simulink model "E_Platoon"  (R2025b)
settings: Solver=FixedStepAuto  StartTime=0.0  StopTime=inf  FixedStep=0.1  RelTol=1e-3
values from neighbouring files (symbols this model uses):
  Battery_Capacity = [1,4500]    [EV_Truck.m]
  battery_SOC_resistance = battery_SOC(:,3)    [EV_Truck.m]
  battery_SOC_SOC = battery_SOC(:,1)    [EV_Truck.m]
  battery_SOC_voltage = battery_SOC(:,2)    [EV_Truck.m]
  motor_efficiency_efficiency = table2array(motor_efficiency(2:height(motor_efficiency),2:width(motor_efficiency)))    [EV_Truck.m]
  motor_efficiency_RPM = table2array(motor_efficiency(2:height(motor_efficiency),1))    [EV_Truck.m]
  motor_efficiency_torque = transpose(motor_efficiency_torque)    [EV_Truck.m]
  motor_RPM_torque = table2array(motor_torque(1:14,1))    [EV_Truck.m]
  motor_torque_RPM = table2array(motor_torque(1:14,2))    [EV_Truck.m]
undefined symbols (not defined in the file or in its folder): Battery_Initial_SOC, DiscIntNeverNeededParam
libraries: simulink x8, BatteryEstimators x4, mpcadaslib x2, slpidlib x2
(part 1 of 2)
settings Model: Creator=geunu6319  LastModifiedBy=geunu6319
settings DataIOCC: SaveFormat=Array  ReturnWorkspaceOutputs=off

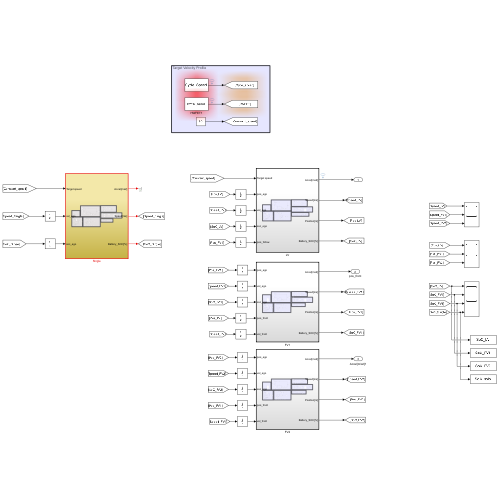
[thumbnail: Simulink's stored preview of the top-level diagram]
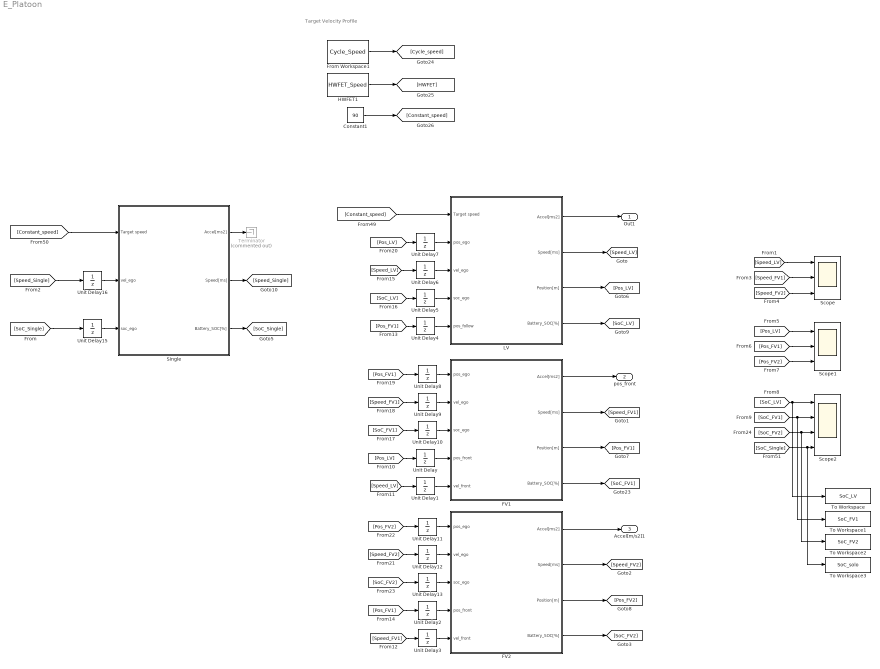
== system E_Platoon ==
  note: Target Velocity Profile
  Constant1 : Constant  Value=90  SampleTime=0
  FV1 : Subsystem  TreatAsAtomicUnit=on
  FV2 : Subsystem  TreatAsAtomicUnit=on
  From Workspace1 : FromWorkspace  VariableName=Cycle_Speed  SampleTime=-1
  HWFET1 : FromWorkspace  VariableName=HWFET_Speed  SampleTime=-1
  LV : Subsystem  TreatAsAtomicUnit=on
  Scope : Scope  NumInputPorts=3
      settings: ActiveDisplayYMinimum=-3.56247  ActiveDisplayYMaximum=3.7997  DataLoggingVariableName=ScopeData5
  Scope1 : Scope  NumInputPorts=3
      settings: ActiveDisplayYMinimum=-50980.76527  ActiveDisplayYMaximum=458458.14542  DataLoggingVariableName=ScopeData6
  Scope2 : Scope  NumInputPorts=4
      settings: ActiveDisplayYMinimum=88.74997  ActiveDisplayYMaximum=101.25001
  Single : Subsystem  TreatAsAtomicUnit=on
  Terminator : Terminator  Commented=on
  To Workspace : ToWorkspace  VariableName=SoC_LV  SaveFormat=Timeseries  SampleTime=-1
  To Workspace1 : ToWorkspace  VariableName=SoC_FV1  SaveFormat=Timeseries  SampleTime=-1
  To Workspace2 : ToWorkspace  VariableName=SoC_FV2  SaveFormat=Timeseries  SampleTime=-1
  To Workspace3 : ToWorkspace  VariableName=SoC_solo  SaveFormat=Timeseries  SampleTime=-1
  Unit Delay{,1..13,15..16} (16 alike) : UnitDelay  SampleTime=-1  HasFrameUpgradeWarning=on
  Out1 : Outport
  pos_front : Outport  Port=2
  Accel[m/s2]1 : Outport  Port=3
  wires:
  LV/2(Speed[ms]) -> [Speed_LV]
  [Pos_LV] -> Scope1/1
  Unit Delay2/1 -> FV2/4(pos_front)
  Unit Delay5/1 -> LV/4(soc_ego)
  [SoC_FV1] -> Unit Delay10/1
  [Speed_LV] -> Unit Delay1/1
  Unit Delay15/1 -> Single/3(soc_ego)
  FV1/1(Accel[ms2]) -> pos_front/1
  [Speed_LV] -> Scope/1
  [SoC_Single] -> To Workspace3/1, Scope2/4
  LV/4(Battery_SOC[%]) -> [SoC_LV]
  Single/1(Accel[ms2]) -> Terminator/1
  [Speed_FV1] -> Unit Delay3/1
  [Constant_speed] -> LV/1(Target speed)
  [Pos_FV1] -> Scope1/2
  Unit Delay16/1 -> Single/2(vel_ego)
  [Pos_LV] -> Unit Delay7/1
  [SoC_FV2] -> To Workspace2/1, Scope2/3
  Constant1/1 -> [Constant_speed]
  Unit Delay6/1 -> LV/3(vel_ego)
  Unit Delay3/1 -> FV2/5(vel_front)
  [Speed_FV1] -> Scope/2
  [Speed_FV2] -> Unit Delay12/1
  Unit Delay11/1 -> FV2/1(pos_ego)
  FV2/4(Battery_SOC[%]) -> [SoC_FV2]
  FV2/2(Speed[ms]) -> [Speed_FV2]
  [Speed_Single] -> Unit Delay16/1
  FV2/3(Position[m]) -> [Pos_FV2]
  [SoC_Single] -> Unit Delay15/1
  Unit Delay12/1 -> FV2/2(vel_ego)
  [Pos_FV2] -> Unit Delay11/1
  Unit Delay4/1 -> LV/5(pos_follow)
  LV/3(Position[m]) -> [Pos_LV]
  [Speed_FV2] -> Scope/3
  Unit Delay13/1 -> FV2/3(soc_ego)
  Unit Delay1/1 -> FV1/5(vel_front)
  [Speed_LV] -> Unit Delay6/1
  [Speed_FV1] -> Unit Delay9/1
  FV2/1(Accel[ms2]) -> Accel[m/s2]1/1
  From Workspace1/1 -> [Cycle_speed]
  [Pos_FV1] -> Unit Delay4/1
  FV1/4(Battery_SOC[%]) -> [SoC_FV1]
  LV/1(Accel[ms2]) -> Out1/1
  [Pos_LV] -> Unit Delay/1
  [SoC_LV] -> To Workspace/1, Scope2/1
  FV1/3(Position[m]) -> [Pos_FV1]
  Single/2(Speed[ms]) -> [Speed_Single]
  [Pos_FV2] -> Scope1/3
  Single/3(Battery_SOC[%]) -> [SoC_Single]
  Unit Delay9/1 -> FV1/2(vel_ego)
  [Pos_FV1] -> Unit Delay2/1
  Unit Delay8/1 -> FV1/1(pos_ego)
  [Pos_FV1] -> Unit Delay8/1
  HWFET1/1 -> [HWFET]
  Unit Delay10/1 -> FV1/3(soc_ego)
  [SoC_FV2] -> Unit Delay13/1
  Unit Delay7/1 -> LV/2(pos_ego)
  [Constant_speed] -> Single/1(Target speed)
  [SoC_FV1] -> To Workspace1/1, Scope2/2
  Unit Delay/1 -> FV1/4(pos_front)
  [SoC_LV] -> Unit Delay5/1
  FV1/2(Speed[ms]) -> [Speed_FV1]

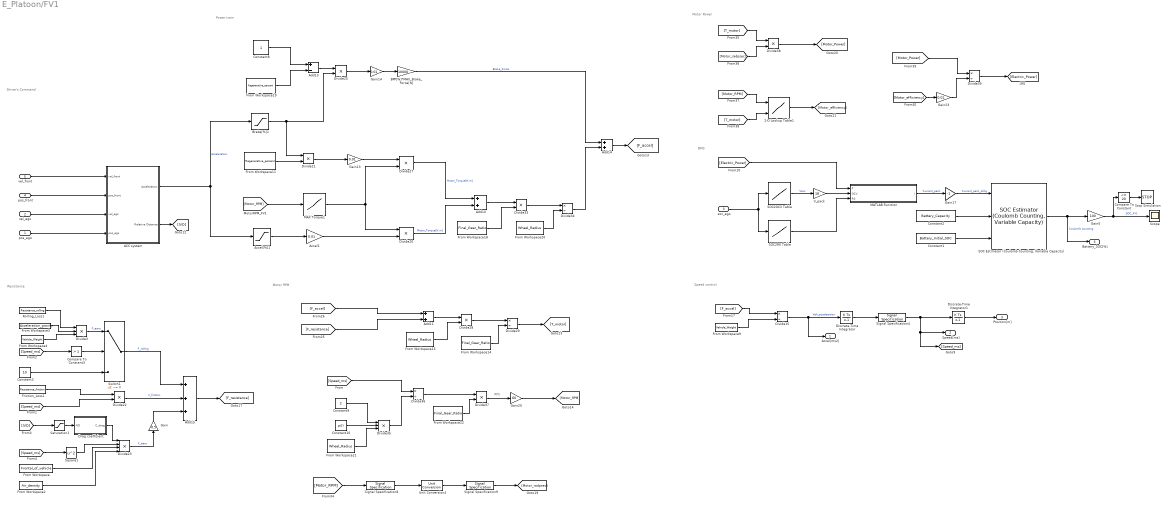
== system E_Platoon/FV1 ==
  note: Driver's Command
  note: Motor RPM
  note: Motor Power
  note: Power train
  note: RPS
  note: Resistance
  note: Speed control
  note: BMS
  pos_ego : Inport
  vel_ego : Inport  Port=2
  soc_ego : Inport  Port=3
  pos_front : Inport  Port=4
  vel_front : Inport  Port=5
  2-D Lookup Table1 : Lookup_n-D  BreakpointsForDimension1=motor_efficiency_RPM  BreakpointsForDimension2=motor_efficiency_torque  Table=motor_efficiency_efficiency  RemoveProtectionInput=on  InternalRulePriority=Speed  RndMeth=Simplest
      settings: InputPortMap=u0,u1
  ACC system : Subsystem
  Accel1 : Gain  Gain=0.01
  Accel[%]1 : Saturate  UpperLimit=100  LowerLimit=0
  Add10 : Sum
  Add11 : Sum
  Add13 : Sum  Inputs=+-
  Add14 : Sum
  Add15 : Sum  Inputs=+++
  BPP[%]*MAX_Brake_Force[N] : Gain  Gain=10000
  Brake[%]1 : Saturate  UpperLimit=0  LowerLimit=-100
  Compare To Constant : simulink/Logic and Bit Operations/Compare To Constant  relop=<=  const=20  OutDataTypeStr=boolean
  Compare To Constant3 : simulink/Logic and Bit Operations/Compare To Constant  relop=>  const=1  OutDataTypeStr=boolean
  Constant1 : Constant  Value=Battery_Initial_SOC
  Constant10 : Constant  Value=pi()
  Constant2 : Constant  Value=Battery_Capacity
  Constant3 : Constant  Value=10
  Constant8 : Constant
  Constant9 : Constant  Value=2
  Discrete-Time Integrator : DiscreteIntegrator  SampleTime=-1  ICPrevOutput=DiscIntNeverNeededParam  ICPrevScaledInput=DiscIntNeverNeededParam
  Discrete-Time Integrator1 : DiscreteIntegrator  SampleTime=-1  ICPrevOutput=DiscIntNeverNeededParam  ICPrevScaledInput=DiscIntNeverNeededParam
  Divide{15,29,34,36,39} (5 alike) : Product  Inputs=*/
  Divide{20..22,25,27..28,33,37..38} (9 alike) : Product  Inputs=**
  Divide23 : Product  Inputs=****
  Divide3 : Product  Inputs=***
  Divide35 : Product  Inputs=***
  Drag coefficient : MATLAB Function  TreatAsAtomicUnit=on
  Friction_Loss1 : FromWorkspace  VariableName=Resistance_friction  SampleTime=0.01
  From Workspace : FromWorkspace  VariableName=Frontal_of_vehicle  SampleTime=0.01
  From Workspace11 : FromWorkspace  VariableName=Regenerative_percent  SampleTime=0.01
  From Workspace14 : FromWorkspace  VariableName=Final_Gear_Ratio  SampleTime=0.01
  From Workspace15 : FromWorkspace  VariableName=Wheel_Radius  SampleTime=0.01
  From Workspace18 : FromWorkspace  VariableName=Final_Gear_Ratio  SampleTime=0.01
  From Workspace19 : FromWorkspace  VariableName=Regenerative_percent  SampleTime=0.01
  From Workspace2 : FromWorkspace  VariableName=Air_density  SampleTime=0.01
  From Workspace20 : FromWorkspace  VariableName=Wheel_Radius  SampleTime=0.01
  From Workspace21 : FromWorkspace  VariableName=Wheel_Radius  SampleTime=0.01
  From Workspace22 : FromWorkspace  VariableName=Final_Gear_Ratio  SampleTime=0.01
  From Workspace3 : FromWorkspace  VariableName=Acceleration_gravity  SampleTime=0.01
  From Workspace4 : FromWorkspace  VariableName=Vehicle_Weight  SampleTime=0.01
  From Workspace9 : FromWorkspace  VariableName=Vehicle_Weight  SampleTime=0.01
  Gain : Gain  Gain=0.5
  Gain13 : Gain  Gain=0.01
  Gain14 : Gain  Gain=0.01
  Gain17 : Gain  Gain=-1
  Gain20 : Gain  Gain=60
  Gain23 : Gain  Gain=0.01
  Gain5 : Gain  Gain=100
  MATLAB Function : MATLAB Function  TreatAsAtomicUnit=on
  MAX Torque1 : Lookup_n-D  NumberOfTableDimensions=1  BreakpointsForDimension1=motor_RPM_torque  Table=motor_torque_RPM  RemoveProtectionInput=on  InternalRulePriority=Speed  RndMeth=Simplest
  Rolling_Loss1 : FromWorkspace  VariableName=Resistance_rolling  SampleTime=0.01
  "SOC Estimator (Coulomb Counting, Variable Capacity)" : BatteryEstimators/SOC Estimator (Coulomb Counting, Variable Capacity)  CurrentInputPartition=on  Ts=1  DataType=Inherit: auto
      settings: LibrarySourceBlock=|
      | batt_sl_lib/Estimators/SOC Estimator
      | (Coulomb Counting, Variable Capacity)
  SOC2OCV Table : Lookup_n-D  NumberOfTableDimensions=1  BreakpointsForDimension1=battery_SOC_SOC  Table=battery_SOC_voltage  ExtrapMethod=Clip  RemoveProtectionInput=on  UseLastTableValue=on  InternalRulePriority=Speed  RndMeth=Simplest
  SOC2R0 Table : Lookup_n-D  NumberOfTableDimensions=1  BreakpointsForDimension1=battery_SOC_SOC  Table=battery_SOC_resistance  RemoveProtectionInput=on  InternalRulePriority=Speed  RndMeth=Simplest
  Saturation1 : Saturate  UpperLimit=100  LowerLimit=0
  Scope : Scope
      settings: DataLoggingVariableName=ScopeData2
  Signal Specification4 : SignalSpecification  Unit=m/s
  Signal Specification8 : SignalSpecification  Unit=rpm
  Signal Specification9 : SignalSpecification  Unit=rad/s
  Square1 : Math  Operator=square
  Stop Simulation : Stop
  Switch1 : Switch  Criteria=u2 ~= 0  SaturateOnIntegerOverflow=off  InputSameDT=off
  Unit Conversion4 : UnitConversion
  V_pack : Gain  Gain=18
  Accel[ms2] : Outport
  Speed[ms] : Outport  Port=2
  Position[m] : Outport  Port=3
  Battery_SOC[%] : Outport  Port=4
  wires:
  vel_front/1 -> ACC system/1(vel_front)
  pos_front/1 -> ACC system/2(pos_front)
  ACC system/2(Relative Distance) -> [IVD]
  From Workspace15/1 -> Divide28/2
  Divide28/1 -> Divide29/1
  From Workspace14/1 -> Divide29/2
  Divide37/1 -> Gain20/1
  Divide36/1 -> Divide37/1
  From Workspace21/1 -> Divide35/3
  Add10/1 -> Divide33/1
  Unit Conversion4/1 -> Signal Specification9/1
  Gain14/1 -> BPP[%]*MAX_Brake_Force[N]/1
  Signal Specification9/1 -> [Motor_radpsec]
  MAX Torque1/1 -> Divide27/2, Divide20/1
  [Motor_RPM] -> MAX Torque1/1
  Divide35/1 -> Divide36/2
  [Motor_RPM] -> Signal Specification8/1
  Gain13/1 -> Divide27/1
  Divide39/1 -> [Electric_Power]
  Divide34/1 -> Add14/2
  Accel[%]1/1 -> Accel1/1
  [Motor_efficiency] -> Gain23/1
  Brake[%]1/1 -> Divide25/2, Divide21/1
  [Motor_RPM] -> 2-D Lookup Table1/1
  Divide25/1 -> Gain14/1
  Constant9/1 -> Divide35/1
  Add13/1 -> Divide25/1
  Divide20/1 -> Add10/2  "Motor_Torque[N.m]"
  [T_motor] -> Divide38/1
  Divide27/1 -> Add10/1  "Motor_Torque[N.m]"
  Divide33/1 -> Divide34/1
  Add14/1 -> [F_accel]
  From Workspace18/1 -> Divide33/2
  From Workspace20/1 -> Divide34/2
  BPP[%]*MAX_Brake_Force[N]/1 -> Add14/1  "Brake_Force"
  Divide38/1 -> [Motor_Power]
  [F_accel] -> Add11/1
  Constant10/1 -> Divide35/2
  [Motor_Power] -> Divide39/1
  [Motor_radpsec] -> Divide38/2
  Gain20/1 -> [Motor_RPM]
  Divide21/1 -> Gain13/1
  [Speed_ms] -> Divide36/1
  Constant8/1 -> Add13/1
  Signal Specification8/1 -> Unit Conversion4/1
  Accel1/1 -> Divide20/2
  From Workspace19/1 -> Add13/2
  From Workspace11/1 -> Divide21/2
  2-D Lookup Table1/1 -> [Motor_efficiency]
  From Workspace22/1 -> Divide37/2
  Gain23/1 -> Divide39/2
  Divide29/1 -> [T_motor]
  [T_motor] -> 2-D Lookup Table1/2
  Add11/1 -> Divide28/1
  [F_resistance] -> Add11/2
  ACC system/1(Acceleration) -> Accel[%]1/1, Brake[%]1/1  "Acceleration"
  From Workspace3/1 -> Divide3/2
  From Workspace/1 -> Divide23/3
  Gain/1 -> Add15/3
  From Workspace2/1 -> Divide23/4
  Divide3/1 -> Switch1/1  "F_aero"
  Divide23/1 -> Gain/1  "F_aero"
  From Workspace4/1 -> Divide3/3
  Saturation1/1 -> Drag coefficient/1(IVD)
  Add15/1 -> [F_resistance]
  Friction_Loss1/1 -> Divide22/1
  Drag coefficient/1(C_drag) -> Divide23/1
  Rolling_Loss1/1 -> Divide3/1
  Compare To Constant3/1 -> Switch1/2
  Square1/1 -> Divide23/2
  Constant3/1 -> Switch1/3
  [IVD] -> Saturation1/1
  [Speed_ms] -> Square1/1
  [Speed_ms] -> Divide22/2
  [Speed_ms] -> Compare To Constant3/1
  Divide22/1 -> Add15/2  "F_friction"
  Switch1/1 -> Add15/1  "F_rolling"
  pos_ego/1 -> ACC system/4(pos_ego)
  vel_ego/1 -> ACC system/3(vel_ego)
  Signal Specification4/1 -> Discrete-Time Integrator1/1, Speed[ms]/1, [Speed_ms]
  Divide15/1 -> Discrete-Time Integrator/1, Accel[ms2]/1  "Veh_acceleartion"
  From Workspace9/1 -> Divide15/2
  Discrete-Time Integrator1/1 -> Position[m]/1
  [F_accel] -> Divide15/1
  Discrete-Time Integrator/1 -> Signal Specification4/1
  Constant1/1 -> "SOC Estimator (Coulomb Counting, Variable Capacity)"/3
  "SOC Estimator (Coulomb Counting, Variable Capacity)"/1 -> Battery_SOC[%]/1, Gain5/1  "Coulomb counting"
  Constant2/1 -> "SOC Estimator (Coulomb Counting, Variable Capacity)"/2
  MATLAB Function/1(I) -> Gain17/1  "Current_pack"
  soc_ego/1 -> SOC2R0 Table/1, SOC2OCV Table/1
  [Electric_Power] -> MATLAB Function/1(P)
  V_pack/1 -> MATLAB Function/2(OCV)
  Gain17/1 -> "SOC Estimator (Coulomb Counting, Variable Capacity)"/1  "Current_pack_dchg"
  Gain5/1 -> Compare To Constant/1, Scope/1  "SOC_FV1"
  Compare To Constant/1 -> Stop Simulation/1
  SOC2R0 Table/1 -> MATLAB Function/3(R0)
  SOC2OCV Table/1 -> V_pack/1  "Vsoc"

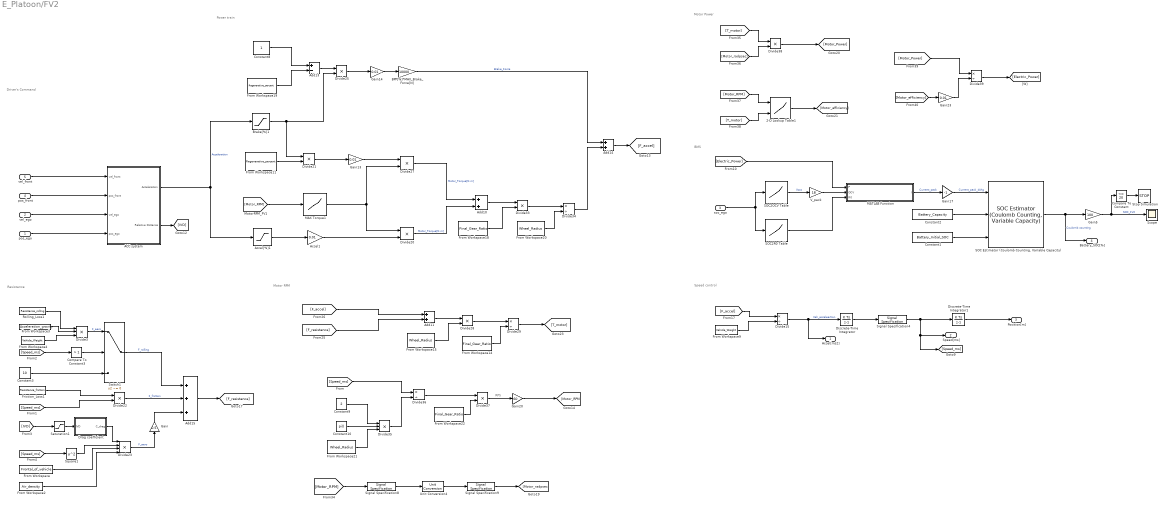
== system E_Platoon/FV2 ==
  note: Driver's Command
  note: Motor RPM
  note: Motor Power
  note: Power train
  note: RPS
  note: Resistance
  note: Speed control
  note: BMS
  pos_ego : Inport
  vel_ego : Inport  Port=2
  soc_ego : Inport  Port=3
  pos_front : Inport  Port=4
  vel_front : Inport  Port=5
  2-D Lookup Table1 : Lookup_n-D  BreakpointsForDimension1=motor_efficiency_RPM  BreakpointsForDimension2=motor_efficiency_torque  Table=motor_efficiency_efficiency  RemoveProtectionInput=on  InternalRulePriority=Speed  RndMeth=Simplest
      settings: InputPortMap=u0,u1
  ACC system : Subsystem
  Accel1 : Gain  Gain=0.01
  Accel[%]1 : Saturate  UpperLimit=100  LowerLimit=0
  Add10 : Sum
  Add11 : Sum
  Add13 : Sum  Inputs=+-
  Add14 : Sum
  Add15 : Sum  Inputs=+++
  BPP[%]*MAX_Brake_Force[N] : Gain  Gain=10000
  Brake[%]1 : Saturate  UpperLimit=0  LowerLimit=-100
  Compare To Constant : simulink/Logic and Bit Operations/Compare To Constant  relop=<=  const=20  OutDataTypeStr=boolean
  Compare To Constant3 : simulink/Logic and Bit Operations/Compare To Constant  relop=>  const=1  OutDataTypeStr=boolean
  Constant1 : Constant  Value=Battery_Initial_SOC
  Constant10 : Constant  Value=pi()
  Constant2 : Constant  Value=Battery_Capacity
  Constant3 : Constant  Value=10
  Constant8 : Constant
  Constant9 : Constant  Value=2
  Discrete-Time Integrator : DiscreteIntegrator  SampleTime=-1  ICPrevOutput=DiscIntNeverNeededParam  ICPrevScaledInput=DiscIntNeverNeededParam
  Discrete-Time Integrator1 : DiscreteIntegrator  SampleTime=-1  ICPrevOutput=DiscIntNeverNeededParam  ICPrevScaledInput=DiscIntNeverNeededParam
  Divide{15,29,34,36,39} (5 alike) : Product  Inputs=*/
  Divide{20..22,25,27..28,33,37..38} (9 alike) : Product  Inputs=**
  Divide23 : Product  Inputs=****
  Divide3 : Product  Inputs=***
  Divide35 : Product  Inputs=***
  Drag coefficient : MATLAB Function  TreatAsAtomicUnit=on
  Friction_Loss1 : FromWorkspace  VariableName=Resistance_friction  SampleTime=0.01
  From Workspace : FromWorkspace  VariableName=Frontal_of_vehicle  SampleTime=0.01
  From Workspace11 : FromWorkspace  VariableName=Regenerative_percent  SampleTime=0.01
  From Workspace14 : FromWorkspace  VariableName=Final_Gear_Ratio  SampleTime=0.01
  From Workspace15 : FromWorkspace  VariableName=Wheel_Radius  SampleTime=0.01
  From Workspace18 : FromWorkspace  VariableName=Final_Gear_Ratio  SampleTime=0.01
  From Workspace19 : FromWorkspace  VariableName=Regenerative_percent  SampleTime=0.01
  From Workspace2 : FromWorkspace  VariableName=Air_density  SampleTime=0.01
  From Workspace20 : FromWorkspace  VariableName=Wheel_Radius  SampleTime=0.01
  From Workspace21 : FromWorkspace  VariableName=Wheel_Radius  SampleTime=0.01
  From Workspace22 : FromWorkspace  VariableName=Final_Gear_Ratio  SampleTime=0.01
  From Workspace3 : FromWorkspace  VariableName=Acceleration_gravity  SampleTime=0.01
  From Workspace4 : FromWorkspace  VariableName=Vehicle_Weight  SampleTime=0.01
  From Workspace9 : FromWorkspace  VariableName=Vehicle_Weight  SampleTime=0.01
  Gain : Gain  Gain=0.5
  Gain13 : Gain  Gain=0.01
  Gain14 : Gain  Gain=0.01
  Gain17 : Gain  Gain=-1
  Gain20 : Gain  Gain=60
  Gain23 : Gain  Gain=0.01
  Gain5 : Gain  Gain=100
  MATLAB Function : MATLAB Function  TreatAsAtomicUnit=on
  MAX Torque1 : Lookup_n-D  NumberOfTableDimensions=1  BreakpointsForDimension1=motor_RPM_torque  Table=motor_torque_RPM  RemoveProtectionInput=on  InternalRulePriority=Speed  RndMeth=Simplest
  Rolling_Loss1 : FromWorkspace  VariableName=Resistance_rolling  SampleTime=0.01
  "SOC Estimator (Coulomb Counting, Variable Capacity)" : BatteryEstimators/SOC Estimator (Coulomb Counting, Variable Capacity)  CurrentInputPartition=on  Ts=1  DataType=Inherit: auto
      settings: LibrarySourceBlock=|
      | batt_sl_lib/Estimators/SOC Estimator
      | (Coulomb Counting, Variable Capacity)
  SOC2OCV Table : Lookup_n-D  NumberOfTableDimensions=1  BreakpointsForDimension1=battery_SOC_SOC  Table=battery_SOC_voltage  ExtrapMethod=Clip  RemoveProtectionInput=on  UseLastTableValue=on  InternalRulePriority=Speed  RndMeth=Simplest
  SOC2R0 Table : Lookup_n-D  NumberOfTableDimensions=1  BreakpointsForDimension1=battery_SOC_SOC  Table=battery_SOC_resistance  RemoveProtectionInput=on  InternalRulePriority=Speed  RndMeth=Simplest
  Saturation1 : Saturate  UpperLimit=100  LowerLimit=0
  Scope : Scope
      settings: DataLoggingVariableName=ScopeData3
  Signal Specification4 : SignalSpecification  Unit=m/s
  Signal Specification8 : SignalSpecification  Unit=rpm
  Signal Specification9 : SignalSpecification  Unit=rad/s
  Square1 : Math  Operator=square
  Stop Simulation : Stop
  Switch1 : Switch  Criteria=u2 ~= 0  SaturateOnIntegerOverflow=off  InputSameDT=off
  Unit Conversion4 : UnitConversion
  V_pack : Gain  Gain=18
  Accel[ms2] : Outport
  Speed[ms] : Outport  Port=2
  Position[m] : Outport  Port=3
  Battery_SOC[%] : Outport  Port=4
  wires:
  vel_front/1 -> ACC system/1(vel_front)
  pos_front/1 -> ACC system/2(pos_front)
  ACC system/2(Relative Distance) -> [IVD]
  From Workspace15/1 -> Divide28/2
  Divide28/1 -> Divide29/1
  From Workspace14/1 -> Divide29/2
  Divide37/1 -> Gain20/1
  Divide36/1 -> Divide37/1
  From Workspace21/1 -> Divide35/3
  Add10/1 -> Divide33/1
  Unit Conversion4/1 -> Signal Specification9/1
  Gain14/1 -> BPP[%]*MAX_Brake_Force[N]/1
  Signal Specification9/1 -> [Motor_radpsec]
  MAX Torque1/1 -> Divide27/2, Divide20/1
  [Motor_RPM] -> MAX Torque1/1
  Divide35/1 -> Divide36/2
  [Motor_RPM] -> Signal Specification8/1
  Gain13/1 -> Divide27/1
  Divide39/1 -> [Electric_Power]
  Divide34/1 -> Add14/2
  Accel[%]1/1 -> Accel1/1
  [Motor_efficiency] -> Gain23/1
  Brake[%]1/1 -> Divide25/2, Divide21/1
  [Motor_RPM] -> 2-D Lookup Table1/1
  Divide25/1 -> Gain14/1
  Constant9/1 -> Divide35/1
  Add13/1 -> Divide25/1
  Divide20/1 -> Add10/2  "Motor_Torque[N.m]"
  [T_motor] -> Divide38/1
  Divide27/1 -> Add10/1  "Motor_Torque[N.m]"
  Divide33/1 -> Divide34/1
  Add14/1 -> [F_accel]
  From Workspace18/1 -> Divide33/2
  From Workspace20/1 -> Divide34/2
  BPP[%]*MAX_Brake_Force[N]/1 -> Add14/1  "Brake_Force"
  Divide38/1 -> [Motor_Power]
  [F_accel] -> Add11/1
  Constant10/1 -> Divide35/2
  [Motor_Power] -> Divide39/1
  [Motor_radpsec] -> Divide38/2
  Gain20/1 -> [Motor_RPM]
  Divide21/1 -> Gain13/1
  [Speed_ms] -> Divide36/1
  Constant8/1 -> Add13/1
  Signal Specification8/1 -> Unit Conversion4/1
  Accel1/1 -> Divide20/2
  From Workspace19/1 -> Add13/2
  From Workspace11/1 -> Divide21/2
  2-D Lookup Table1/1 -> [Motor_efficiency]
  From Workspace22/1 -> Divide37/2
  Gain23/1 -> Divide39/2
  Divide29/1 -> [T_motor]
  [T_motor] -> 2-D Lookup Table1/2
  Add11/1 -> Divide28/1
  [F_resistance] -> Add11/2
  ACC system/1(Acceleration) -> Accel[%]1/1, Brake[%]1/1  "Acceleration"
  From Workspace3/1 -> Divide3/2
  From Workspace/1 -> Divide23/3
  Gain/1 -> Add15/3
  From Workspace2/1 -> Divide23/4
  Divide3/1 -> Switch1/1  "F_aero"
  Divide23/1 -> Gain/1  "F_aero"
  From Workspace4/1 -> Divide3/3
  Saturation1/1 -> Drag coefficient/1(IVD)
  Add15/1 -> [F_resistance]
  Friction_Loss1/1 -> Divide22/1
  Drag coefficient/1(C_drag) -> Divide23/1
  Rolling_Loss1/1 -> Divide3/1
  Compare To Constant3/1 -> Switch1/2
  Square1/1 -> Divide23/2
  Constant3/1 -> Switch1/3
  [IVD] -> Saturation1/1
  [Speed_ms] -> Square1/1
  [Speed_ms] -> Divide22/2
  [Speed_ms] -> Compare To Constant3/1
  Divide22/1 -> Add15/2  "F_friction"
  Switch1/1 -> Add15/1  "F_rolling"
  pos_ego/1 -> ACC system/4(pos_ego)
  vel_ego/1 -> ACC system/3(vel_ego)
  Signal Specification4/1 -> Discrete-Time Integrator1/1, Speed[ms]/1, [Speed_ms]
  Divide15/1 -> Discrete-Time Integrator/1, Accel[ms2]/1  "Veh_acceleartion"
  From Workspace9/1 -> Divide15/2
  Discrete-Time Integrator1/1 -> Position[m]/1
  [F_accel] -> Divide15/1
  Discrete-Time Integrator/1 -> Signal Specification4/1
  Constant1/1 -> "SOC Estimator (Coulomb Counting, Variable Capacity)"/3
  "SOC Estimator (Coulomb Counting, Variable Capacity)"/1 -> Battery_SOC[%]/1, Gain5/1  "Coulomb counting"
  Constant2/1 -> "SOC Estimator (Coulomb Counting, Variable Capacity)"/2
  MATLAB Function/1(I) -> Gain17/1  "Current_pack"
  soc_ego/1 -> SOC2R0 Table/1, SOC2OCV Table/1
  [Electric_Power] -> MATLAB Function/1(P)
  V_pack/1 -> MATLAB Function/2(OCV)
  Gain17/1 -> "SOC Estimator (Coulomb Counting, Variable Capacity)"/1  "Current_pack_dchg"
  Gain5/1 -> Compare To Constant/1, Scope/1  "SOC_FV2"
  Compare To Constant/1 -> Stop Simulation/1
  SOC2R0 Table/1 -> MATLAB Function/3(R0)
  SOC2OCV Table/1 -> V_pack/1  "Vsoc"

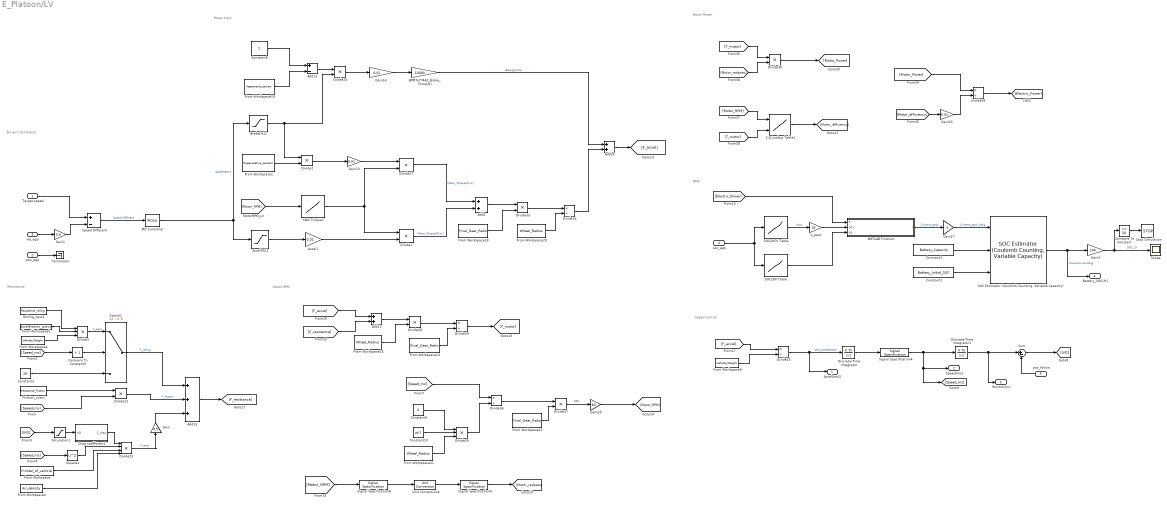
== system E_Platoon/LV ==
  note: Speed control
  note: Driver's Command
  note: BMS
  note: RPS
  note: Power train
  note: Resistance
  note: Motor RPM
  note: Motor Power
  Target speed : Inport
  pos_ego : Inport  Port=2
  vel_ego : Inport  Port=3
  soc_ego : Inport  Port=4
  pos_follow : Inport  Port=5
  2-D Lookup Table1 : Lookup_n-D  BreakpointsForDimension1=motor_efficiency_RPM  BreakpointsForDimension2=motor_efficiency_torque  Table=motor_efficiency_efficiency  RemoveProtectionInput=on  InternalRulePriority=Speed  RndMeth=Simplest
      settings: InputPortMap=u0,u1
  Accel1 : Gain  Gain=0.01
  Accel[%]1 : Saturate  UpperLimit=100  LowerLimit=0
  Add1 : Sum
  Add11 : Sum
  Add13 : Sum  Inputs=+-
  Add14 : Sum
  Add15 : Sum  Inputs=+++
  BPP[%]*MAX_Brake_Force[N] : Gain  Gain=10000
  Brake[%]1 : Saturate  UpperLimit=0  LowerLimit=-100
  Compare To Constant : simulink/Logic and Bit Operations/Compare To Constant  relop=<=  const=20  OutDataTypeStr=boolean
  Compare To Constant3 : simulink/Logic and Bit Operations/Compare To Constant  relop=>  const=1  OutDataTypeStr=boolean
  Constant1 : Constant  Value=Battery_Initial_SOC
  Constant10 : Constant  Value=pi()
  Constant2 : Constant  Value=Battery_Capacity
  Constant3 : Constant  Value=10
  Constant8 : Constant
  Constant9 : Constant  Value=2
  Discrete-Time Integrator : DiscreteIntegrator  SampleTime=-1  ICPrevOutput=DiscIntNeverNeededParam  ICPrevScaledInput=DiscIntNeverNeededParam
  Discrete-Time Integrator1 : DiscreteIntegrator  SampleTime=-1  ICPrevOutput=DiscIntNeverNeededParam  ICPrevScaledInput=DiscIntNeverNeededParam
  Divide{1..2,22,25,27..28,33,37..38} (9 alike) : Product  Inputs=**
  Divide{15,29,34,36,39} (5 alike) : Product  Inputs=*/
  Divide23 : Product  Inputs=****
  Divide3 : Product  Inputs=***
  Divide35 : Product  Inputs=***
  Drag coefficient1 : MATLAB Function  TreatAsAtomicUnit=on
  Friction_Loss1 : FromWorkspace  VariableName=Resistance_friction  SampleTime=0.01
  From Workspace : FromWorkspace  VariableName=Frontal_of_vehicle  SampleTime=0.01
  From Workspace1 : FromWorkspace  VariableName=Regenerative_percent  SampleTime=0.01
  From Workspace14 : FromWorkspace  VariableName=Final_Gear_Ratio  SampleTime=0.01
  From Workspace15 : FromWorkspace  VariableName=Wheel_Radius  SampleTime=0.01
  From Workspace18 : FromWorkspace  VariableName=Final_Gear_Ratio  SampleTime=0.01
  From Workspace19 : FromWorkspace  VariableName=Regenerative_percent  SampleTime=0.01
  From Workspace2 : FromWorkspace  VariableName=Air_density  SampleTime=0.01
  From Workspace20 : FromWorkspace  VariableName=Wheel_Radius  SampleTime=0.01
  From Workspace21 : FromWorkspace  VariableName=Wheel_Radius  SampleTime=0.01
  From Workspace22 : FromWorkspace  VariableName=Final_Gear_Ratio  SampleTime=0.01
  From Workspace3 : FromWorkspace  VariableName=Acceleration_gravity  SampleTime=0.01
  From Workspace4 : FromWorkspace  VariableName=Vehicle_Weight  SampleTime=0.01
  From Workspace9 : FromWorkspace  VariableName=Vehicle_Weight  SampleTime=0.01
  Gain : Gain  Gain=0.5
  Gain1 : Gain  Gain=3.6
  Gain13 : Gain  Gain=0.01
  Gain14 : Gain  Gain=0.01
  Gain17 : Gain  Gain=-1
  Gain20 : Gain  Gain=60
  Gain23 : Gain  Gain=0.01
  Gain5 : Gain  Gain=100
  MATLAB Function : MATLAB Function  TreatAsAtomicUnit=on
  MAX Torque1 : Lookup_n-D  NumberOfTableDimensions=1  BreakpointsForDimension1=motor_RPM_torque  Table=motor_torque_RPM  RemoveProtectionInput=on  InternalRulePriority=Speed  RndMeth=Simplest
  PID Controller : slpidlib/PID Controller  Controller=PID  Form=Parallel  TimeDomain=Discrete-time  UseExternalTs=off  SampleTime=-1  IntegratorMethod=Forward Euler  FilterMethod=Forward Euler  ControllerParametersSource=internal  P=100  I=0.01  UseKiTs=off  D=0.0001  UseExternalDerivativeSource=off  N=10  UseFilter=on  TunerSelectOption=Transfer Function Based (PID Tuner App)  InitialConditionSource=internal  InitialConditionForIntegrator=0  InitialConditionForFilter=0  DifferentiatorICPrevScaledInput=0  ExternalReset=none  TrackingMode=off  Kt=1  LimitOutput=off  SatLimitsSource=internal  UpperSaturationLimit=inf  LowerSaturationLimit=-inf  LinearizeAsGain=on  AntiWindupMode=none  Kb=1  LimitIntegrator=off  UpperIntegratorSaturationLimit=inf  LowerIntegratorSaturationLimit=-inf  POutMin=[]  POutMax=[]  IOutMin=[]  IOutMax=[]  DOutMin=[]  DOutMax=[]  NOutMin=[]  NOutMax=[]  SumOutMin=[]  SumOutMax=[]  SaturationOutMin=[]  SaturationOutMax=[]  PParamMin=[]  PParamMax=[]  IParamMin=[]  IParamMax=[]  DParamMin=[]  DParamMax=[]  NParamMin=[]  NParamMax=[]  KbParamMin=[]  KbParamMax=[]  KtParamMin=[]  KtParamMax=[]  KbOutMin=[]  KbOutMax=[]  KtOutMin=[]  KtOutMax=[]  IntegratorOutMin=[]  IntegratorOutMax=[]  FilterOutMin=[]  FilterOutMax=[]  SumI1OutMin=[]  SumI1OutMax=[]  SumI2OutMin=[]  SumI2OutMax=[]  SumI3OutMin=[]  SumI3OutMax=[]  SumI4OutMin=[]  SumI4OutMax=[]  SumDOutMin=[]  SumDOutMax=[]  DifferentiatorOutMin=[]  DifferentiatorOutMax=[]  FilterDiffOutCoefMin=[]  FilterDiffOutCoefMax=[]  ReciprocalOutMin=[]  ReciprocalOutMax=[]  SumDenOutMin=[]  SumDenOutMax=[]  SumNumOutMin=[]  SumNumOutMax=[]  DivideOutMin=[]  DivideOutMax=[]  UdiffTsProdOutMin=[]  UdiffTsProdOutMax=[]  NTsProdOutMin=[]  NTsProdOutMax=[]  UintegralTsProdOutMin=[]  UintegralTsProdOutMax=[]  UngainTsProdOutMin=[]  UngainTsProdOutMax=[]  ClampingZeroOutDataTypeStr=Inherit: Inherit via back propagation  ClampingZeroOutMin=[]  ClampingZeroOutMax=[]  FilterDenConstantOutDataTypeStr=Inherit: Inherit via back propagation  FilterDenConstantOutMin=[]  FilterDenConstantOutMax=[]  PCopyOutDataTypeStr=Inherit: Inherit via back propagation  PCopyOutMin=[]  PCopyOutMax=[]  NCopyOutDataTypeStr=Inherit: Inherit via back propagation  NCopyOutMin=[]  NCopyOutMax=[]  IntegratorContinuousStateAttributes=''  IntegratorStateMustResolveToSignalObject=off  IntegratorRTWStateStorageClass=Auto  FilterContinuousStateAttributes=''  FilterStateMustResolveToSignalObject=off  FilterRTWStateStorageClass=Auto  ParallelPVariant=InternalParameters  IdealPVariant=Disabled  IVariant=InternalParameters  DVariant=InternalParameters  IntegratorVariant=Discrete  SatVariant=Disabled  AWVariant=Passthrough  PCopyVariant=Disabled  TRVariant=Disabled  FdbkBlocksVariant=Forward  IdealPFdbkVariant=Disabled  SatFdbkVariant=Disabled  DerivativeFilterVariant=ForwardEulerFilter  NVariant=InternalParameters  NCopyVariant=Disabled  FilterICVariant=InternalICsFilter  IntegratorICVariant=InternalICs  ExternalResetVariant=Disabled  TRSumVariant=Passthrough  SumFdbkVariant=Disabled  SumVariant=Sum_PID  TsampFilterVariant=InternalTs  TsampNgainVariant=Passthrough  TsampIntegralVariant=Disabled_SignalSpec  ExternalSaturationOutDataTypeStr=Inherit: Same as second input  DerivativeSourceVariant=ErrorSignal  PreIntVariant=InternalPreInt
  Rolling_Loss1 : FromWorkspace  VariableName=Resistance_rolling  SampleTime=0.01
  "SOC Estimator (Coulomb Counting, Variable Capacity)" : BatteryEstimators/SOC Estimator (Coulomb Counting, Variable Capacity)  CurrentInputPartition=on  Ts=1  DataType=Inherit: auto
      settings: LibrarySourceBlock=|
      | batt_sl_lib/Estimators/SOC Estimator
      | (Coulomb Counting, Variable Capacity)
  SOC2OCV Table : Lookup_n-D  NumberOfTableDimensions=1  BreakpointsForDimension1=battery_SOC_SOC  Table=battery_SOC_voltage  ExtrapMethod=Clip  RemoveProtectionInput=on  UseLastTableValue=on  InternalRulePriority=Speed  RndMeth=Simplest
  SOC2R0 Table : Lookup_n-D  NumberOfTableDimensions=1  BreakpointsForDimension1=battery_SOC_SOC  Table=battery_SOC_resistance  RemoveProtectionInput=on  InternalRulePriority=Speed  RndMeth=Simplest
  Saturation1 : Saturate  UpperLimit=100  LowerLimit=0
  Scope : Scope
  Signal Specification4 : SignalSpecification  Unit=m/s
  Signal Specification8 : SignalSpecification  Unit=rpm
  Signal Specification9 : SignalSpecification  Unit=rad/s
  Speed Different : Sum  Inputs=+-
  Square1 : Math  Operator=square
  Stop Simulation : Stop
  Sum : Sum  Inputs=|+-
  Switch1 : Switch  Criteria=u2 ~= 0  SaturateOnIntegerOverflow=off  InputSameDT=off
  Terminator : Terminator
  Unit Conversion4 : UnitConversion
  V_pack : Gain  Gain=18
  Accel[ms2] : Outport
  Speed[ms] : Outport  Port=2
  Position[m] : Outport  Port=3
  Battery_SOC[%] : Outport  Port=4
  wires:
  Discrete-Time Integrator1/1 -> Sum/1, Position[m]/1
  From Workspace9/1 -> Divide15/2
  Divide15/1 -> Discrete-Time Integrator/1, Accel[ms2]/1  "Veh_acceleartion"
  pos_follow/1 -> Sum/2
  Discrete-Time Integrator/1 -> Signal Specification4/1
  Signal Specification4/1 -> Discrete-Time Integrator1/1, Speed[ms]/1, [Speed_ms]
  PID Controller/1 -> Brake[%]1/1, Accel[%]1/1  "Acceleration"
  Speed Different/1 -> PID Controller/1  "Speed Different"
  Target speed/1 -> Speed Different/1
  vel_ego/1 -> Gain1/1
  soc_ego/1 -> SOC2R0 Table/1, SOC2OCV Table/1
  MATLAB Function/1(I) -> Gain17/1  "Current_pack"
  Gain5/1 -> Compare To Constant/1, Scope/1  "SOC_LV"
  Sum/1 -> [IVD]
  Divide28/1 -> Divide29/1
  From Workspace20/1 -> Divide34/2
  Add1/1 -> Divide33/1
  [T_motor] -> Divide38/1
  Divide29/1 -> [T_motor]
  Signal Specification9/1 -> [Motor_radpsec]
  [IVD] -> Saturation1/1
  Gain20/1 -> [Motor_RPM]
  Add13/1 -> Divide25/1
  Divide39/1 -> [Electric_Power]
  Add14/1 -> [F_accel]
  [Speed_ms] -> Divide22/2
  [F_resistance] -> Add11/2
  Divide1/1 -> Add1/2  "Motor_Torque[N.m]"
  From Workspace14/1 -> Divide29/2
  Divide23/1 -> Gain/1  "F_aero"
  Brake[%]1/1 -> Divide25/2, Divide2/1
  Unit Conversion4/1 -> Signal Specification9/1
  From Workspace21/1 -> Divide35/3
  Divide35/1 -> Divide36/2
  [Motor_RPM] -> 2-D Lookup Table1/1
  Gain23/1 -> Divide39/2
  Compare To Constant3/1 -> Switch1/2
  Divide37/1 -> Gain20/1
  Divide34/1 -> Add14/2
  BPP[%]*MAX_Brake_Force[N]/1 -> Add14/1  "Brake_Force"
  From Workspace/1 -> Divide23/3
  From Workspace22/1 -> Divide37/2
  Constant9/1 -> Divide35/1
  [Motor_efficiency] -> Gain23/1
  Constant10/1 -> Divide35/2
  [Speed_ms] -> Square1/1
  Add11/1 -> Divide28/1
  Square1/1 -> Divide23/2
  2-D Lookup Table1/1 -> [Motor_efficiency]
  Gain14/1 -> BPP[%]*MAX_Brake_Force[N]/1
  From Workspace19/1 -> Add13/2
  Add15/1 -> [F_resistance]
  Friction_Loss1/1 -> Divide22/1
  [Motor_RPM] -> Signal Specification8/1
  Drag coefficient1/1(C_drag) -> Divide23/1
  [Motor_radpsec] -> Divide38/2
  From Workspace1/1 -> Divide2/2
  Accel[%]1/1 -> Accel1/1
  Constant8/1 -> Add13/1
  Divide36/1 -> Divide37/1
  [Motor_Power] -> Divide39/1
  MAX Torque1/1 -> Divide27/2, Divide1/1
  Accel1/1 -> Divide1/2
  Divide33/1 -> Divide34/1
  [F_accel] -> Add11/1
  [T_motor] -> 2-D Lookup Table1/2
  Rolling_Loss1/1 -> Divide3/1
  Divide27/1 -> Add1/1  "Motor_Torque[N.m]"
  Saturation1/1 -> Drag coefficient1/1(IVD)
  Switch1/1 -> Add15/1  "F_rolling"
  From Workspace15/1 -> Divide28/2
  Gain13/1 -> Divide27/1
  Constant3/1 -> Switch1/3
  Divide25/1 -> Gain14/1
  Divide22/1 -> Add15/2  "F_friction"
  Divide2/1 -> Gain13/1
  Divide38/1 -> [Motor_Power]
  [Motor_RPM] -> MAX Torque1/1
  Signal Specification8/1 -> Unit Conversion4/1
  From Workspace18/1 -> Divide33/2
  [Speed_ms] -> Divide36/1
  [F_accel] -> Divide15/1
  [Speed_ms] -> Compare To Constant3/1
  Gain/1 -> Add15/3
  From Workspace2/1 -> Divide23/4
  From Workspace3/1 -> Divide3/2
  From Workspace4/1 -> Divide3/3
  Divide3/1 -> Switch1/1  "F_aero"
  Compare To Constant/1 -> Stop Simulation/1
  Gain1/1 -> Speed Different/2
  pos_ego/1 -> Terminator/1
  "SOC Estimator (Coulomb Counting, Variable Capacity)"/1 -> Battery_SOC[%]/1, Gain5/1  "Coulomb counting"
  Gain17/1 -> "SOC Estimator (Coulomb Counting, Variable Capacity)"/1  "Current_pack_dchg"
  Constant1/1 -> "SOC Estimator (Coulomb Counting, Variable Capacity)"/3
  [Electric_Power] -> MATLAB Function/1(P)
  V_pack/1 -> MATLAB Function/2(OCV)
  SOC2R0 Table/1 -> MATLAB Function/3(R0)
  SOC2OCV Table/1 -> V_pack/1  "Vsoc"
  Constant2/1 -> "SOC Estimator (Coulomb Counting, Variable Capacity)"/2

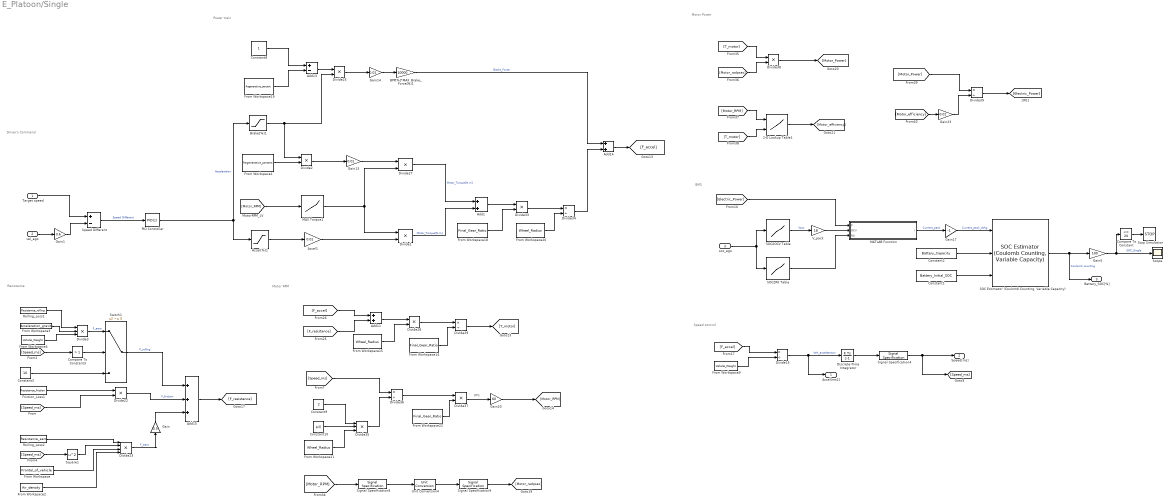
== system E_Platoon/Single ==
  note: Speed control
  note: Driver's Command
  note: RPS
  note: Power train
  note: Resistance
  note: Motor RPM
  note: Motor Power
  note: BMS
  Target speed : Inport
  vel_ego : Inport  Port=2
  soc_ego : Inport  Port=3
  2-D Lookup Table1 : Lookup_n-D  BreakpointsForDimension1=motor_efficiency_RPM  BreakpointsForDimension2=motor_efficiency_torque  Table=motor_efficiency_efficiency  InternalRulePriority=Speed  RndMeth=Simplest
      settings: InputPortMap=u0,u1
  Accel1 : Gain  Gain=0.01
  Accel[%]1 : Saturate  UpperLimit=100  LowerLimit=0
  Add1 : Sum
  Add11 : Sum
  Add13 : Sum  Inputs=+-
  Add14 : Sum
  Add15 : Sum  Inputs=+++
  BPP[%]*MAX_Brake_Force[N]1 : Gain  Gain=10000
  Brake[%]1 : Saturate  UpperLimit=0  LowerLimit=-100
  Compare To Constant : simulink/Logic and Bit Operations/Compare To Constant  relop=<=  const=20  OutDataTypeStr=boolean
  Compare To Constant3 : simulink/Logic and Bit Operations/Compare To Constant  relop=>  const=1  OutDataTypeStr=boolean
  Constant1 : Constant  Value=Battery_Initial_SOC
  Constant10 : Constant  Value=pi()
  Constant2 : Constant  Value=Battery_Capacity
  Constant3 : Constant  Value=10
  Constant8 : Constant
  Constant9 : Constant  Value=2
  Discrete-Time Integrator : DiscreteIntegrator  SampleTime=-1  ICPrevOutput=DiscIntNeverNeededParam  ICPrevScaledInput=DiscIntNeverNeededParam
  Divide{1..2,22,25,27..28,33,37..38} (9 alike) : Product  Inputs=**
  Divide{15,29,34,36,39} (5 alike) : Product  Inputs=*/
  Divide23 : Product  Inputs=****
  Divide3 : Product  Inputs=***
  Divide35 : Product  Inputs=***
  Friction_Loss1 : FromWorkspace  VariableName=Resistance_friction
  From Workspace : FromWorkspace  VariableName=Frontal_of_vehicle
  From Workspace1 : FromWorkspace  VariableName=Regenerative_percent
  From Workspace14 : FromWorkspace  VariableName=Final_Gear_Ratio
  From Workspace15 : FromWorkspace  VariableName=Wheel_Radius
  From Workspace18 : FromWorkspace  VariableName=Final_Gear_Ratio
  From Workspace19 : FromWorkspace  VariableName=Regenerative_percent
  From Workspace2 : FromWorkspace  VariableName=Air_density
  From Workspace20 : FromWorkspace  VariableName=Wheel_Radius
  From Workspace21 : FromWorkspace  VariableName=Wheel_Radius
  From Workspace22 : FromWorkspace  VariableName=Final_Gear_Ratio
  From Workspace3 : FromWorkspace  VariableName=Acceleration_gravity
  From Workspace4 : FromWorkspace  VariableName=Vehicle_Weight
  From Workspace9 : FromWorkspace  VariableName=Vehicle_Weight
  Gain : Gain  Gain=0.5
  Gain1 : Gain  Gain=3.6
  Gain13 : Gain  Gain=0.01
  Gain14 : Gain  Gain=0.01
  Gain17 : Gain  Gain=-1
  Gain20 : Gain  Gain=60
  Gain23 : Gain  Gain=0.01
  Gain5 : Gain  Gain=100
  MATLAB Function : MATLAB Function  TreatAsAtomicUnit=on
  MAX Torque1 : Lookup_n-D  NumberOfTableDimensions=1  BreakpointsForDimension1=motor_RPM_torque  Table=motor_torque_RPM  InternalRulePriority=Speed  RndMeth=Simplest
  PID Controller : slpidlib/PID Controller  Controller=PID  Form=Parallel  TimeDomain=Discrete-time  UseExternalTs=off  SampleTime=-1  IntegratorMethod=Forward Euler  FilterMethod=Forward Euler  ControllerParametersSource=internal  P=100  I=0.01  UseKiTs=off  D=0.0001  UseExternalDerivativeSource=off  N=10  UseFilter=on  TunerSelectOption=Transfer Function Based (PID Tuner App)  InitialConditionSource=internal  InitialConditionForIntegrator=0  InitialConditionForFilter=0  DifferentiatorICPrevScaledInput=0  ExternalReset=none  TrackingMode=off  Kt=1  LimitOutput=off  SatLimitsSource=internal  UpperSaturationLimit=inf  LowerSaturationLimit=-inf  LinearizeAsGain=on  AntiWindupMode=none  Kb=1  LimitIntegrator=off  UpperIntegratorSaturationLimit=inf  LowerIntegratorSaturationLimit=-inf  POutMin=[]  POutMax=[]  IOutMin=[]  IOutMax=[]  DOutMin=[]  DOutMax=[]  NOutMin=[]  NOutMax=[]  SumOutMin=[]  SumOutMax=[]  SaturationOutMin=[]  SaturationOutMax=[]  PParamMin=[]  PParamMax=[]  IParamMin=[]  IParamMax=[]  DParamMin=[]  DParamMax=[]  NParamMin=[]  NParamMax=[]  KbParamMin=[]  KbParamMax=[]  KtParamMin=[]  KtParamMax=[]  KbOutMin=[]  KbOutMax=[]  KtOutMin=[]  KtOutMax=[]  IntegratorOutMin=[]  IntegratorOutMax=[]  FilterOutMin=[]  FilterOutMax=[]  SumI1OutMin=[]  SumI1OutMax=[]  SumI2OutMin=[]  SumI2OutMax=[]  SumI3OutMin=[]  SumI3OutMax=[]  SumI4OutMin=[]  SumI4OutMax=[]  SumDOutMin=[]  SumDOutMax=[]  DifferentiatorOutMin=[]  DifferentiatorOutMax=[]  FilterDiffOutCoefMin=[]  FilterDiffOutCoefMax=[]  ReciprocalOutMin=[]  ReciprocalOutMax=[]  SumDenOutMin=[]  SumDenOutMax=[]  SumNumOutMin=[]  SumNumOutMax=[]  DivideOutMin=[]  DivideOutMax=[]  UdiffTsProdOutMin=[]  UdiffTsProdOutMax=[]  NTsProdOutMin=[]  NTsProdOutMax=[]  UintegralTsProdOutMin=[]  UintegralTsProdOutMax=[]  UngainTsProdOutMin=[]  UngainTsProdOutMax=[]  ClampingZeroOutDataTypeStr=Inherit: Inherit via back propagation  ClampingZeroOutMin=[]  ClampingZeroOutMax=[]  FilterDenConstantOutDataTypeStr=Inherit: Inherit via back propagation  FilterDenConstantOutMin=[]  FilterDenConstantOutMax=[]  PCopyOutDataTypeStr=Inherit: Inherit via back propagation  PCopyOutMin=[]  PCopyOutMax=[]  NCopyOutDataTypeStr=Inherit: Inherit via back propagation  NCopyOutMin=[]  NCopyOutMax=[]  IntegratorContinuousStateAttributes=''  IntegratorStateMustResolveToSignalObject=off  IntegratorRTWStateStorageClass=Auto  FilterContinuousStateAttributes=''  FilterStateMustResolveToSignalObject=off  FilterRTWStateStorageClass=Auto  ParallelPVariant=InternalParameters  IdealPVariant=Disabled  IVariant=InternalParameters  DVariant=InternalParameters  IntegratorVariant=Discrete  SatVariant=Disabled  AWVariant=Passthrough  PCopyVariant=Disabled  TRVariant=Disabled  FdbkBlocksVariant=Forward  IdealPFdbkVariant=Disabled  SatFdbkVariant=Disabled  DerivativeFilterVariant=ForwardEulerFilter  NVariant=InternalParameters  NCopyVariant=Disabled  FilterICVariant=InternalICsFilter  IntegratorICVariant=InternalICs  ExternalResetVariant=Disabled  TRSumVariant=Passthrough  SumFdbkVariant=Disabled  SumVariant=Sum_PID  TsampFilterVariant=InternalTs  TsampNgainVariant=Passthrough  TsampIntegralVariant=Disabled_SignalSpec  ExternalSaturationOutDataTypeStr=Inherit: Same as second input  DerivativeSourceVariant=ErrorSignal  PreIntVariant=InternalPreInt
  Rolling_Loss1 : FromWorkspace  VariableName=Resistance_rolling
  Rolling_Loss2 : FromWorkspace  VariableName=Resistance_aero
  "SOC Estimator (Coulomb Counting, Variable Capacity)" : BatteryEstimators/SOC Estimator (Coulomb Counting, Variable Capacity)  CurrentInputPartition=on  Ts=1  DataType=Inherit: auto
      settings: LibrarySourceBlock=|
      | batt_sl_lib/Estimators/SOC Estimator
      | (Coulomb Counting, Variable Capacity)
  SOC2OCV Table : Lookup_n-D  NumberOfTableDimensions=1  BreakpointsForDimension1=battery_SOC_SOC  Table=battery_SOC_voltage  ExtrapMethod=Clip  RemoveProtectionInput=on  UseLastTableValue=on  InternalRulePriority=Speed  RndMeth=Simplest
  SOC2R0 Table : Lookup_n-D  NumberOfTableDimensions=1  BreakpointsForDimension1=battery_SOC_SOC  Table=battery_SOC_resistance  RemoveProtectionInput=on  InternalRulePriority=Speed  RndMeth=Simplest
  Scope : Scope
      settings: DataLoggingVariableName=ScopeData4
  Signal Specification4 : SignalSpecification  Unit=m/s
  Signal Specification8 : SignalSpecification  Unit=rpm
  Signal Specification9 : SignalSpecification  Unit=rad/s
  Speed Different : Sum  Inputs=+-
  Square1 : Math  Operator=square
  Stop Simulation : Stop
  Switch1 : Switch  Criteria=u2 ~= 0  SaturateOnIntegerOverflow=off  InputSameDT=off
  Unit Conversion4 : UnitConversion
  V_pack : Gain  Gain=18
  Accel[ms2] : Outport
  Speed[ms] : Outport  Port=2
  Battery_SOC[%] : Outport  Port=3
  wires:
  From Workspace9/1 -> Divide15/2
  Divide15/1 -> Discrete-Time Integrator/1, Accel[ms2]/1  "Veh_acceleartion"
  Discrete-Time Integrator/1 -> Signal Specification4/1
  Signal Specification4/1 -> [Speed_ms], Speed[ms]/1
  PID Controller/1 -> Brake[%]1/1, Accel[%]1/1  "Acceleration"
  Speed Different/1 -> PID Controller/1  "Speed Different"
  Target speed/1 -> Speed Different/1
  vel_ego/1 -> Gain1/1
  Divide28/1 -> Divide29/1
  From Workspace20/1 -> Divide34/2
  Add1/1 -> Divide33/1
  [T_motor] -> Divide38/1
  Divide29/1 -> [T_motor]
  Signal Specification9/1 -> [Motor_radpsec]
  Gain20/1 -> [Motor_RPM]
  Add13/1 -> Divide25/1
  Divide39/1 -> [Electric_Power]
  Add14/1 -> [F_accel]
  [Speed_ms] -> Divide22/2
  [F_resistance] -> Add11/2
  Divide1/1 -> Add1/2  "Motor_Torque[N.m]"
  From Workspace14/1 -> Divide29/2
  Divide23/1 -> Gain/1  "F_aero"
  Brake[%]1/1 -> Divide25/2, Divide2/1
  Unit Conversion4/1 -> Signal Specification9/1
  From Workspace21/1 -> Divide35/3
  Divide35/1 -> Divide36/2
  [Motor_RPM] -> 2-D Lookup Table1/1
  Gain23/1 -> Divide39/2
  Compare To Constant3/1 -> Switch1/2
  Divide37/1 -> Gain20/1
  Divide34/1 -> Add14/2
  BPP[%]*MAX_Brake_Force[N]1/1 -> Add14/1  "Brake_Force"
  From Workspace/1 -> Divide23/3
  From Workspace22/1 -> Divide37/2
  Constant9/1 -> Divide35/1
  [Motor_efficiency] -> Gain23/1
  Constant10/1 -> Divide35/2
  [Speed_ms] -> Square1/1
  Add11/1 -> Divide28/1
  Square1/1 -> Divide23/2
  2-D Lookup Table1/1 -> [Motor_efficiency]
  Gain14/1 -> BPP[%]*MAX_Brake_Force[N]1/1
  From Workspace19/1 -> Add13/2
  Add15/1 -> [F_resistance]
  Friction_Loss1/1 -> Divide22/1
  [Motor_RPM] -> Signal Specification8/1
  Rolling_Loss2/1 -> Divide23/1
  [Motor_radpsec] -> Divide38/2
  From Workspace1/1 -> Divide2/2
  Accel[%]1/1 -> Accel1/1
  Constant8/1 -> Add13/1
  Divide36/1 -> Divide37/1
  [Motor_Power] -> Divide39/1
  MAX Torque1/1 -> Divide27/2, Divide1/1
  Accel1/1 -> Divide1/2
  Divide33/1 -> Divide34/1
  [F_accel] -> Add11/1
  [T_motor] -> 2-D Lookup Table1/2
  Rolling_Loss1/1 -> Divide3/1
  Divide27/1 -> Add1/1  "Motor_Torque[N.m]"
  Switch1/1 -> Add15/1  "F_rolling"
  From Workspace15/1 -> Divide28/2
  Gain13/1 -> Divide27/1
  Constant3/1 -> Switch1/3
  Divide25/1 -> Gain14/1
  Divide22/1 -> Add15/2  "F_friction"
  Divide2/1 -> Gain13/1
  Divide38/1 -> [Motor_Power]
  [Motor_RPM] -> MAX Torque1/1
  Signal Specification8/1 -> Unit Conversion4/1
  From Workspace18/1 -> Divide33/2
  [Speed_ms] -> Divide36/1
  [F_accel] -> Divide15/1
  [Speed_ms] -> Compare To Constant3/1
  Gain/1 -> Add15/3
  From Workspace2/1 -> Divide23/4
  From Workspace3/1 -> Divide3/2
  From Workspace4/1 -> Divide3/3
  Divide3/1 -> Switch1/1  "F_aero"
  Gain1/1 -> Speed Different/2
  Constant1/1 -> "SOC Estimator (Coulomb Counting, Variable Capacity)"/3
  "SOC Estimator (Coulomb Counting, Variable Capacity)"/1 -> Battery_SOC[%]/1, Gain5/1  "Coulomb counting"
  Constant2/1 -> "SOC Estimator (Coulomb Counting, Variable Capacity)"/2
  MATLAB Function/1(I) -> Gain17/1  "Current_pack"
  soc_ego/1 -> SOC2R0 Table/1, SOC2OCV Table/1
  [Electric_Power] -> MATLAB Function/1(P)
  V_pack/1 -> MATLAB Function/2(OCV)
  Gain17/1 -> "SOC Estimator (Coulomb Counting, Variable Capacity)"/1  "Current_pack_dchg"
  Gain5/1 -> Compare To Constant/1, Scope/1  "SOC_Single"
  Compare To Constant/1 -> Stop Simulation/1
  SOC2R0 Table/1 -> MATLAB Function/3(R0)
  SOC2OCV Table/1 -> V_pack/1  "Vsoc"

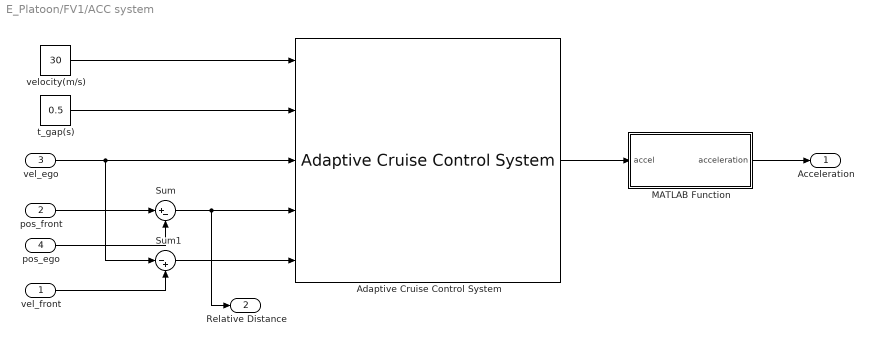
== system E_Platoon/FV1/ACC system ==
  vel_front : Inport
  pos_front : Inport  Port=2
  vel_ego : Inport  Port=3
  pos_ego : Inport  Port=4
  Adaptive Cruise Control System : mpcadaslib/Adaptive Cruise Control System  EgoModel=tf(1,[0.5,1,0])  InitialEgoVelocity=20  DefaultSpacing=20  MaxVelocity=30  MinAcceleration=-3  amin_ext=off  MaxAcceleration=3  amax_ext=off  Ts=0.01  PredictionHorizon=100  ControllerBehavior=0.7  suboptimal=off  maxiter=10  datatypeopt=double  optmode=off  trackmode=off
  MATLAB Function : MATLAB Function  TreatAsAtomicUnit=on
  Sum : Sum  Inputs=|+-
  Sum1 : Sum  Inputs=|-+
  t_gap(s) : Constant  Value=0.5
  velocity(m/s) : Constant  Value=30
  Acceleration : Outport
  Relative Distance : Outport  Port=2
  wires:
  t_gap(s)/1 -> Adaptive Cruise Control System/2
  Sum/1 -> Relative Distance/1, Adaptive Cruise Control System/4
  Sum1/1 -> Adaptive Cruise Control System/5
  velocity(m/s)/1 -> Adaptive Cruise Control System/1
  Adaptive Cruise Control System/1 -> MATLAB Function/1(accel)
  pos_front/1 -> Sum/1
  pos_ego/1 -> Sum/2
  vel_front/1 -> Sum1/2
  vel_ego/1 -> Sum1/1, Adaptive Cruise Control System/3
  MATLAB Function/1(acceleration) -> Acceleration/1

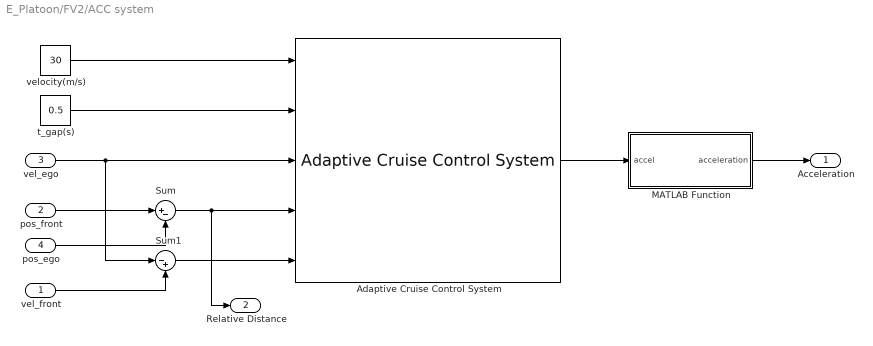
== system E_Platoon/FV2/ACC system ==
  vel_front : Inport
  pos_front : Inport  Port=2
  vel_ego : Inport  Port=3
  pos_ego : Inport  Port=4
  Adaptive Cruise Control System : mpcadaslib/Adaptive Cruise Control System  EgoModel=tf(1,[0.5,1,0])  InitialEgoVelocity=20  DefaultSpacing=20  MaxVelocity=30  MinAcceleration=-3  amin_ext=off  MaxAcceleration=3  amax_ext=off  Ts=0.01  PredictionHorizon=100  ControllerBehavior=0.7  suboptimal=off  maxiter=10  datatypeopt=double  optmode=off  trackmode=off
  MATLAB Function : MATLAB Function  TreatAsAtomicUnit=on
  Sum : Sum  Inputs=|+-
  Sum1 : Sum  Inputs=|-+
  t_gap(s) : Constant  Value=0.5
  velocity(m/s) : Constant  Value=30
  Acceleration : Outport
  Relative Distance : Outport  Port=2
  wires:
  t_gap(s)/1 -> Adaptive Cruise Control System/2
  Sum/1 -> Relative Distance/1, Adaptive Cruise Control System/4
  Sum1/1 -> Adaptive Cruise Control System/5
  velocity(m/s)/1 -> Adaptive Cruise Control System/1
  Adaptive Cruise Control System/1 -> MATLAB Function/1(accel)
  pos_front/1 -> Sum/1
  pos_ego/1 -> Sum/2
  vel_front/1 -> Sum1/2
  vel_ego/1 -> Sum1/1, Adaptive Cruise Control System/3
  MATLAB Function/1(acceleration) -> Acceleration/1

== matlab function E_Platoon/FV1/MATLAB Function ==
  data: P input; OCV input; R0 input; I output
function I = current_from_power(P, OCV, R0)
% 1-R battery model:
%   Vt = OCV - R0*I
%   P  = Vt*I = I*(OCV - R0*I)
% => R0*I^2 - OCV*I + P = 0
%   I = (OCV - sqrt(OCV^2 - 4*R0*P)) / (2*R0)
%
%   P>0 -> I>0 (discharge)
%   P<0 -> I<0 (regen/charge)

epsR = 1e-12;
epsV = 1e-6;
R0  = max(R0, epsR);
OCV = max(OCV, epsV);

% Discriminant
D = OCV*OCV - 4*R0*P;

% If D < 0, the requested P is infeasible under this simple model.
% Clamp to 0 to avoid complex values (simple fallback).
if D < 0
    D = 0;
end

% Minus-branch current
I = (OCV - sqrt(D)) / (2*R0);

% Safety
if ~isfinite(I)
    I = 0;
end
end

== matlab function E_Platoon/LV/Drag coefficient1 ==
  data: IVD input; C_drag output
function C_drag = fcn(IVD)
a = -0.1012;
b = -0.1002;
c = 0.6441;

C_drag = a * exp(b * (IVD-8)) + c;

== matlab function E_Platoon/Single/MATLAB Function ==
  data: P input; OCV input; R0 input; I output
function I = current_from_power(P, OCV, R0)
% 1-R battery model:
%   Vt = OCV - R0*I
%   P  = Vt*I = I*(OCV - R0*I)
% => R0*I^2 - OCV*I + P = 0
%   I = (OCV - sqrt(OCV^2 - 4*R0*P)) / (2*R0)
%
%   P>0 -> I>0 (discharge)
%   P<0 -> I<0 (regen/charge)

epsR = 1e-12;
epsV = 1e-6;
R0  = max(R0, epsR);
OCV = max(OCV, epsV);

% Discriminant
D = OCV*OCV - 4*R0*P;

% If D < 0, the requested P is infeasible under this simple model.
% Clamp to 0 to avoid complex values (simple fallback).
if D < 0
    D = 0;
end

% Minus-branch current
I = (OCV - sqrt(D)) / (2*R0);

% Safety
if ~isfinite(I)
    I = 0;
end
end

== matlab function E_Platoon/FV2/MATLAB Function ==
  data: P input; OCV input; R0 input; I output
function I = current_from_power(P, OCV, R0)
% 1-R battery model:
%   Vt = OCV - R0*I
%   P  = Vt*I = I*(OCV - R0*I)
% => R0*I^2 - OCV*I + P = 0
%   I = (OCV - sqrt(OCV^2 - 4*R0*P)) / (2*R0)
%
%   P>0 -> I>0 (discharge)
%   P<0 -> I<0 (regen/charge)

epsR = 1e-12;
epsV = 1e-6;
R0  = max(R0, epsR);
OCV = max(OCV, epsV);

% Discriminant
D = OCV*OCV - 4*R0*P;

% If D < 0, the requested P is infeasible under this simple model.
% Clamp to 0 to avoid complex values (simple fallback).
if D < 0
    D = 0;
end

% Minus-branch current
I = (OCV - sqrt(D)) / (2*R0);

% Safety
if ~isfinite(I)
    I = 0;
end
end

== matlab function E_Platoon/FV2/ACC system/MATLAB Function ==
  data: accel input; acceleration output
function acceleration  = fcn(accel)

if accel > 0 
    acceleration = (accel * 100)/0.15;
elseif accel < 0 
    acceleration = (accel * 100)/0.33;
else
    acceleration = 0; % accel이 0이거나 NaN일 경우에도 대응
end
